simulink model "RL_TTS3_Controller_Blank_NLC_valve_E"  (R2019b)
settings: Solver=FixedStepAuto  StartTime=0.0  StopTime=600  FixedStep=0.01  RelTol=1e-3
PostLoadFcn:
  | if any(exist('dsrtsu_mdlpostloadfcn', 'file') ~= 0), dsrtsu_mdlpostloadfcn('Execute', bdroot); end
values from neighbouring files (symbols this model uses):
  Ts = 0.1    [RL_TTS3_Controller_Blank.mat]
libraries: simulink x2
settings Model: DSRTSU_INTERNAL_RTI_VER=550  DSRTSU_INTERNAL_RTI_TYPE=rti1104  RTICANMMDATA=struct('GeneralSetupData',struct('modelroot','E:\Will\RemoteLabs\TTS3\HostPC','generalsettings',struct('filesettings',struct('destfolder',struct('Name','RTICANMM_FILES','Check',1),'buildfolder',struct('Name','.','Check',1),'AbsDestfolder',struct('Name','E:\Will\RemoteLabs\TTS3\HostPC\RTICANMM_FILES'),'AbsBuildfolder',struct('Name','E:\Will\RemoteLabs\TTS3\HostPC'))),'options',struct('addpaths',1,'rmpaths',1,'addtrcexclusion',true,'cannavigator',struct('checkmonitoring',0),'show_usrtrc',0,'use_usrtrc',0),'advanced',struct('options',ones(1,100)),'MPSetup',{{}},'RTI',struct('Type','RTI1104','Ver','7.13','Date','02-Nov-2019'),'modelname','TTS3_Controller_Test_OL','block','TTS3_Controller_Test_OL'))  DSRTSU_INTERNAL_RTIFPGA=150  Creator=whendrix  LastModifiedBy=karan
settings OptimizationCC: BlockReduction=off  OptimizeBlockIOStorage=off  BufferReuse=off  GlobalBufferReuse=off  ExpressionFolding=off  LocalBlockOutputs=off  OptimizeDataStoreBuffers=off  BusAssignmentInplaceUpdate=off
settings DebuggingCC: BusObjectLabelMismatch=none
settings HardwareCC: ProdBitPerPointer=32  ProdBitPerSizeT=32  ProdBitPerPtrDiffT=32  ProdLargestAtomicInteger=Integer  ProdEndianess=BigEndian  ProdWordSize=32  ProdHWDeviceType=Custom Processor->Custom  TargetIntDivRoundTo=Zero  TargetEndianess=BigEndian  TargetHWDeviceType=Custom Processor->Custom
settings ModelReferenceCC: ModelReferenceNumInstancesAllowed=Single  ModelReferenceMinAlgLoopOccurrences=on
settings SFSimCC: MATLABDynamicMemAlloc=off  CustomCodeUndefinedFunction=UseInterfaceOnly
settings RTWCC: Description=dSPACE DS1104 Hardware Platform  SystemTargetFile=rti1104.tlc  MakeCommand=make_rti  TemplateMakefile=rti1104.tmf
settings CodeAppCC: MaxIdLength=63
settings STFCustomTargetCC: ParMdlRefBuildCompliant=on  SystemTargetFile=rti1104.tlc
settings GRTTargetCC: TargetLangStandard=C89/C90 (ANSI)  CompOptLevelCompliant=off  ConcurrentExecutionCompliant=off  CombineOutputUpdateFcns=off  MatFileLogging=off  CPPClassGenCompliant=off  UseToolchainInfoCompliant=off

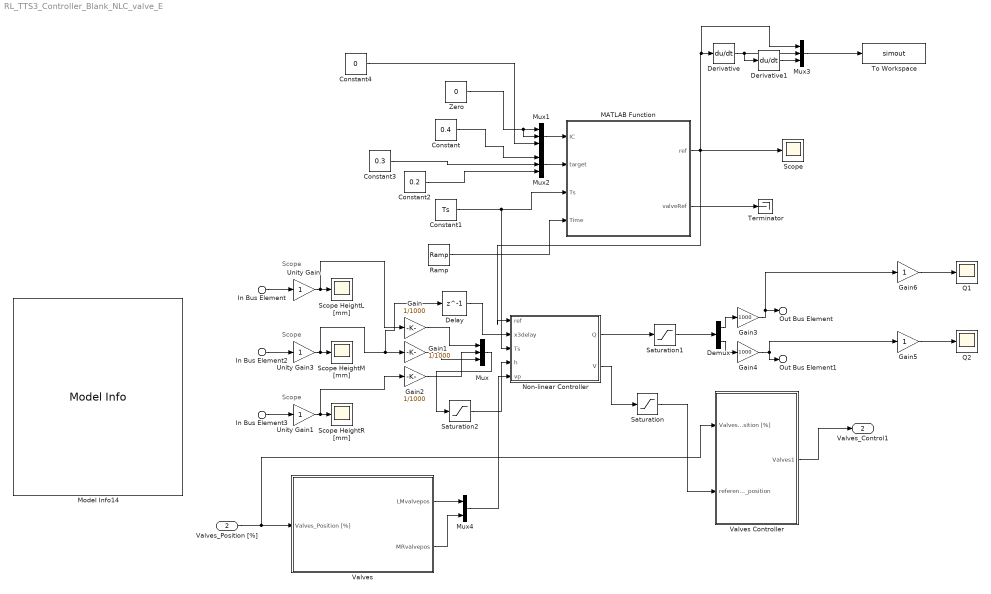
== system RL_TTS3_Controller_Blank_NLC_valve_E ==
  note: Scope
  note: Scope
  note: Scope
  In Bus Element : Inport  PortName=Heights [mm]  Element=Left
  In Bus Element2 : Inport  PortName=Heights [mm]  Element=Middle
  In Bus Element3 : Inport  PortName=Heights [mm]  Element=Right
  Valves_Position [%] : Inport  Port=2  OutDataTypeStr=Bus: ValvesSOCI
  Constant : Constant  Value=0.4
  Constant1 : Constant  Value=Ts
  Constant2 : Constant  Value=0.2
  Constant3 : Constant  Value=0.3
  Constant4 : Constant  Value=0
  Delay : Delay  DelayLength=1
  Demux : Demux  Outputs=2
  Derivative : Derivative
  Derivative1 : Derivative
  Gain : Gain  Gain=1/1000
  Gain1 : Gain  Gain=1/1000
  Gain2 : Gain  Gain=1/1000
  Gain3 : Gain  Gain=1000
  Gain4 : Gain  Gain=1000
  Gain5 : Gain
  Gain6 : Gain
  MATLAB Function : MATLAB Function  TreatAsAtomicUnit=on
  Model Info14 : simulink/Model-Wide Utilities/Model Info  Frame=on  DisplayStringWithTags=|  HorizontalTextAlignment=Left  LeftAlignmentValue=0.02
      | Start model for the "Three Tank"
      | experiment on the "Three Tank" setup.
      | Version: 1.0
      | 
      | 
      | INFORMATION
      | ----------------------
      | 
      | Unity Gain block before Scope is needed for
      | RemoteLabs compatebility. 
      | Do not modify or remove!
      | 
      | Pump range:
      | 0 to 0.102 [l/s]
      | 
      | The 5 Valves are labeled according 
      | to their position:
      | 
      |    LM  MR
      |      X     X
      |  X      X      X
      | LD    MD   RD
      | 
      | L = Left
      | M = Middle
      | R = Right
      | D = Down
  Mux{,1..3} (4 alike) : Mux  Inputs=3
  Mux4 : Mux  Inputs=2
  Non-linear Controller : MATLAB Function  TreatAsAtomicUnit=on
  Q1 : Scope
  Q2 : Scope
  Ramp : simulink/Sources/Ramp  slope=1  start=0  InitialOutput=0
  Saturation : Saturate  UpperLimit=100  LowerLimit=0
  Saturation1 : Saturate  UpperLimit=1.02e-4  LowerLimit=0
  Saturation2 : Saturate  UpperLimit=0.6  LowerLimit=0
  Scope : Scope
  Scope HeightL [mm] : Scope
  Scope HeightM [mm] : Scope
  Scope HeightR [mm] : Scope
  Terminator : Terminator
  To Workspace : ToWorkspace  VariableName=simout  SaveFormat=Timeseries  SampleTime=-1
  Unity Gain : Gain
  Unity Gain1 : Gain
  Unity Gain3 : Gain
  Valves : Subsystem  TreatAsAtomicUnit=on
  Valves Controller : Subsystem
  Zero : Constant  Value=0  OutDataTypeStr=Inherit: Inherit via back propagation
  Out Bus Element : Outport  VectorParamsAs1DForOutWhenUnconnected=off  PortName=Pumps [l/s]  Element=Left
  Out Bus Element1 : Outport  VectorParamsAs1DForOutWhenUnconnected=off  PortName=Pumps [l/s]  Element=Right
  Valves_Control1 : Outport  Port=2  OutDataTypeStr=Bus: ValvesSICO  VectorParamsAs1DForOutWhenUnconnected=off
  wires:
  Unity Gain/1 -> Gain/1, Scope HeightL [mm]/1
  Unity Gain3/1 -> Gain1/1, Delay/1, Scope HeightM [mm]/1
  Unity Gain1/1 -> Gain2/1, Scope HeightR [mm]/1
  In Bus Element/1 -> Unity Gain/1
  In Bus Element2/1 -> Unity Gain3/1
  In Bus Element3/1 -> Unity Gain1/1
  Mux/1 -> Saturation2/1
  Gain2/1 -> Mux/2
  Gain1/1 -> Mux/3
  Gain/1 -> Mux/1
  Saturation1/1 -> Demux/1
  Gain3/1 -> Gain6/1, Out Bus Element/1
  Demux/1 -> Gain3/1
  Demux/2 -> Gain4/1
  Gain4/1 -> Gain5/1, Out Bus Element1/1
  Valves Controller/1(Valves1) -> Valves_Control1/1
  Saturation/1 -> Valves Controller/2("reference_valve_position ")
  Mux1/1 -> MATLAB Function/1(IC)
  Mux3/1 -> To Workspace/1
  Constant/1 -> Mux2/1
  MATLAB Function/1(ref) -> Non-linear Controller/1(ref), Scope/1, Mux3/1, Derivative/1
  Constant4/1 -> Mux1/3
  MATLAB Function/2(valveRef) -> Terminator/1
  Constant3/1 -> Mux2/2
  Zero/1 -> Mux1/2, Mux1/1
  Derivative1/1 -> Mux3/3
  Constant1/1 -> Non-linear Controller/3(Ts), MATLAB Function/3(Ts)
  Constant2/1 -> Mux2/3
  Derivative/1 -> Derivative1/1, Mux3/2
  Mux2/1 -> MATLAB Function/2(target)
  Ramp/1 -> MATLAB Function/4(Time)
  Gain5/1 -> Q2/1
  Gain6/1 -> Q1/1
  Delay/1 -> Non-linear Controller/2(x3delay)
  Non-linear Controller/2(V) -> Saturation/1
  Valves_Position [%]/1 -> Valves Controller/1(Valves_Position [%]), Valves/1(Valves_Position [%])
  Valves/1(LMvalvepos) -> Mux4/1
  Valves/2("MRvalvepos ") -> Mux4/2
  Mux4/1 -> Non-linear Controller/5(vp)
  Non-linear Controller/1(Q) -> Saturation1/1
  Saturation2/1 -> Non-linear Controller/4(h)

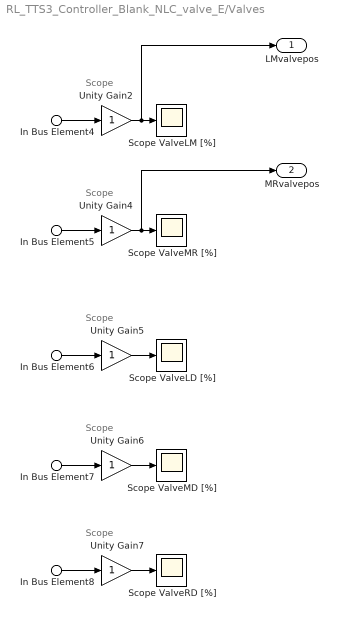
== system RL_TTS3_Controller_Blank_NLC_valve_E/Valves ==
  note: Scope
  note: Scope
  note: Scope
  note: Scope
  note: Scope
  In Bus Element4 : Inport  PortName=Valves_Position [%]  Element=LeftMiddle
  In Bus Element5 : Inport  PortName=Valves_Position [%]  Element=MiddleRight
  In Bus Element6 : Inport  PortName=Valves_Position [%]  Element=LeftDown
  In Bus Element7 : Inport  PortName=Valves_Position [%]  Element=MiddleDown
  In Bus Element8 : Inport  PortName=Valves_Position [%]  Element=RightDown
  Scope ValveLD [%] : Scope
  Scope ValveLM [%] : Scope
  Scope ValveMD [%] : Scope
  Scope ValveMR [%] : Scope
  Scope ValveRD [%] : Scope
  Unity Gain{2,4..7} (5 alike) : Gain
  LMvalvepos : Outport
  "MRvalvepos " : Outport  Port=2
  wires:
  In Bus Element5/1 -> Unity Gain4/1
  In Bus Element4/1 -> Unity Gain2/1
  In Bus Element7/1 -> Unity Gain6/1
  Unity Gain6/1 -> Scope ValveMD [%]/1
  In Bus Element6/1 -> Unity Gain5/1
  In Bus Element8/1 -> Unity Gain7/1
  Unity Gain7/1 -> Scope ValveRD [%]/1
  Unity Gain4/1 -> "MRvalvepos "/1, Scope ValveMR [%]/1
  Unity Gain5/1 -> Scope ValveLD [%]/1
  Unity Gain2/1 -> LMvalvepos/1, Scope ValveLM [%]/1

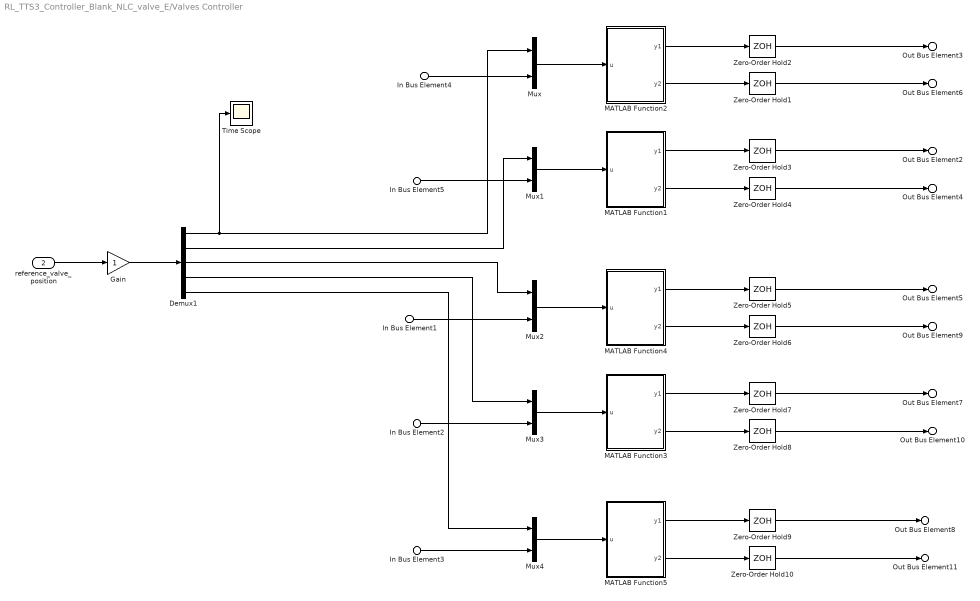
== system RL_TTS3_Controller_Blank_NLC_valve_E/Valves Controller ==
  In Bus Element4 : Inport  PortName=Valves_Position [%]  Element=LeftMiddle
  In Bus Element5 : Inport  PortName=Valves_Position [%]  Element=MiddleRight
  In Bus Element1 : Inport  PortName=Valves_Position [%]  Element=LeftDown
  In Bus Element2 : Inport  PortName=Valves_Position [%]  Element=MiddleDown
  In Bus Element3 : Inport  PortName=Valves_Position [%]  Element=RightDown
  "reference_valve_position " : Inport  Port=2
  Demux1 : Demux  Outputs=5
  Gain : Gain
  MATLAB Function1 : MATLAB Function  TreatAsAtomicUnit=on
  MATLAB Function2 : MATLAB Function  TreatAsAtomicUnit=on
  MATLAB Function3 : MATLAB Function  TreatAsAtomicUnit=on
  MATLAB Function4 : MATLAB Function  TreatAsAtomicUnit=on
  MATLAB Function5 : MATLAB Function  TreatAsAtomicUnit=on
  Mux{,1..4} (5 alike) : Mux  Inputs=2
  Time Scope : Scope
  Zero-Order Hold{1..10} (10 alike) : ZeroOrderHold  SampleTime=0.5
  Out Bus Element8 : Outport  VectorParamsAs1DForOutWhenUnconnected=off  PortName=Valves1  Element=RightDown.Open
  Out Bus Element11 : Outport  VectorParamsAs1DForOutWhenUnconnected=off  PortName=Valves1  Element=RightDown.Close
  Out Bus Element5 : Outport  VectorParamsAs1DForOutWhenUnconnected=off  PortName=Valves1  Element=LeftDown.Open
  Out Bus Element9 : Outport  VectorParamsAs1DForOutWhenUnconnected=off  PortName=Valves1  Element=LeftDown.Close
  Out Bus Element7 : Outport  VectorParamsAs1DForOutWhenUnconnected=off  PortName=Valves1  Element=MiddleDown.Open
  Out Bus Element10 : Outport  VectorParamsAs1DForOutWhenUnconnected=off  PortName=Valves1  Element=MiddleDown.Close
  Out Bus Element2 : Outport  VectorParamsAs1DForOutWhenUnconnected=off  PortName=Valves1  Element=MiddleRight.Open
  Out Bus Element4 : Outport  VectorParamsAs1DForOutWhenUnconnected=off  PortName=Valves1  Element=MiddleRight.Close
  Out Bus Element3 : Outport  VectorParamsAs1DForOutWhenUnconnected=off  PortName=Valves1  Element=LeftMiddle.Open
  Out Bus Element6 : Outport  VectorParamsAs1DForOutWhenUnconnected=off  PortName=Valves1  Element=LeftMiddle.Close
  wires:
  Zero-Order Hold5/1 -> Out Bus Element5/1
  Zero-Order Hold6/1 -> Out Bus Element9/1
  Zero-Order Hold9/1 -> Out Bus Element8/1
  Zero-Order Hold10/1 -> Out Bus Element11/1
  Zero-Order Hold8/1 -> Out Bus Element10/1
  Zero-Order Hold7/1 -> Out Bus Element7/1
  In Bus Element4/1 -> Mux/2
  Mux/1 -> MATLAB Function2/1(u)
  In Bus Element5/1 -> Mux1/2
  Demux1/2 -> Mux1/1
  Zero-Order Hold1/1 -> Out Bus Element6/1
  Zero-Order Hold2/1 -> Out Bus Element3/1
  Demux1/1 -> Time Scope/1, Mux/1
  Mux1/1 -> MATLAB Function1/1(u)
  Zero-Order Hold3/1 -> Out Bus Element2/1
  Zero-Order Hold4/1 -> Out Bus Element4/1
  Mux3/1 -> MATLAB Function3/1(u)
  Demux1/3 -> Mux2/1
  Demux1/4 -> Mux3/1
  In Bus Element2/1 -> Mux3/2
  Mux2/1 -> MATLAB Function4/1(u)
  In Bus Element1/1 -> Mux2/2
  In Bus Element3/1 -> Mux4/2
  Demux1/5 -> Mux4/1
  Mux4/1 -> MATLAB Function5/1(u)
  "reference_valve_position "/1 -> Gain/1
  Gain/1 -> Demux1/1
  MATLAB Function2/1(y1) -> Zero-Order Hold2/1
  MATLAB Function2/2(y2) -> Zero-Order Hold1/1
  MATLAB Function1/1(y1) -> Zero-Order Hold3/1
  MATLAB Function1/2(y2) -> Zero-Order Hold4/1
  MATLAB Function4/1(y1) -> Zero-Order Hold5/1
  MATLAB Function4/2(y2) -> Zero-Order Hold6/1
  MATLAB Function3/1(y1) -> Zero-Order Hold7/1
  MATLAB Function3/2(y2) -> Zero-Order Hold8/1
  MATLAB Function5/1(y1) -> Zero-Order Hold9/1
  MATLAB Function5/2(y2) -> Zero-Order Hold10/1

== matlab function RL_TTS3_Controller_Blank_NLC_valve_E/Valves Controller/MATLAB Function2 ==
  data: u input; y1 output; y2 output
function [y1,y2] = fcn(u)
    if u(2)>u(1)
        y1 = false;
        y2 = true;
    elseif u(1)>u(2)
        y1 = true;
        y2 = false;
    else
        y1 = false;
        y2 = false;
    end
end

== matlab function RL_TTS3_Controller_Blank_NLC_valve_E/Non-linear Controller ==
  data: ref input; x3delay input; Ts input; h input; Q output; V output; vp input
function [Q,V] = fcn(ref,x3delay,Ts,h,vp)

xr = [0.2 0.3 0.25];
x3dot = (h(3)-x3delay)/Ts;
% xr = [ref(1) ref(2) ref(3)];
A = 0.0154; S = 5e-5; g = 9.81;
x1 = h(1); x2 = h(2); x3 = h(3); x4 = vp(1); x5 = vp(2); g = 9.81; 
c1 = 16.1462; c2 = 15.5166; cc = 12/100; cd = 100/99;
x1r = xr(1); x2r = xr(2); x3r = xr(3);

Q = [0 0];
V = zeros(1,5);

u1 = A*(x1r - x1 + (2^(1/2)*S*c1*g^(1/2)*exp(cc*x4)*(x1 - x3))/(A*abs(x1 - x3)^(1/2)*(exp(cc*x4) + 1)));
u2 = A*(x2r - x2 + (2^(1/2)*S*c2*g^(1/2)*exp(cc*x5)*(x2 - x3))/(A*abs(x2 - x3)^(1/2)*(exp(cc*x5) + 1)));
u3 = (2^(1/2)*A*c1*sign(x1 - x3)^2*sign(x2 - x3)^2*exp(cc*x4)*sign(g)*(x1 - x3)*(exp(cc*x4) + 1)^2*(exp(cc*x5) + 1)^4*(x3r - 2*x3dot - x2 + (((2^(1/2)*S*c1*g^(1/2)*exp(cc*x4)*sign(g))/(2*abs(x1 - x3)^(1/2)*(exp(cc*x4) + 1)) + (2^(1/2)*S*c2*g^(1/2)*exp(cc*x5)*sign(g))/(2*abs(x2 - x3)^(1/2)*(exp(cc*x5) + 1)))*((2^(1/2)*S*c1*g^(1/2)*exp(cc*x4)*sign(g)*(x1 - x3))/(abs(x1 - x3)^(1/2)*(exp(cc*x4) + 1)) + (2^(1/2)*S*c2*g^(1/2)*exp(cc*x5)*sign(g)*(x2 - x3))/(abs(x2 - x3)^(1/2)*(exp(cc*x5) + 1))))/A^2 + (S^2*c1^2*g*sign(x1 - x3)*exp(2*cc*x4))/(A^2*(exp(cc*x4) + 1)^2) + (S^2*c2^2*g*sign(x2 - x3)*exp(2*cc*x5))/(A^2*(exp(cc*x5) + 1)^2) + (2^(1/2)*S*c1*cc*cd*g^(1/2)*x4*exp(cc*x4)*sign(g)*(x1 - x3))/(A^2*abs(x1 - x3)^(1/2)*(exp(cc*x4) + 1)^2) + (2^(1/2)*S*c2*cc*cd*g^(1/2)*x5*exp(cc*x5)*sign(g)*(x2 - x3))/(A^2*abs(x2 - x3)^(1/2)*(exp(cc*x5) + 1)^2)))/(2*S*cc*cd*g^(1/2)*abs(x1 - x3)^(1/2)*(6*c1^2*x1*sign(x1 - x3)*exp(2*cc*(x4 + x5)) - 6*c1^2*x3*sign(x1 - x3)*exp(2*cc*(x4 + x5)) + 6*c2^2*x2*sign(x2 - x3)*exp(2*cc*(x4 + x5)) - 6*c2^2*x3*sign(x2 - x3)*exp(2*cc*(x4 + x5)) + c1^2*x1*sign(x1 - x3)*exp(2*cc*x4) - c1^2*x3*sign(x1 - x3)*exp(2*cc*x4) + c2^2*x2*sign(x2 - x3)*exp(2*cc*x5) - c2^2*x3*sign(x2 - x3)*exp(2*cc*x5) + 4*c1^2*x1*sign(x1 - x3)*exp(cc*(2*x4 + x5)) + c1^2*x1*sign(x1 - x3)*exp(2*cc*(x4 + 2*x5)) - 4*c1^2*x3*sign(x1 - x3)*exp(cc*(2*x4 + x5)) + 4*c2^2*x2*sign(x2 - x3)*exp(cc*(x4 + 2*x5)) - c1^2*x3*sign(x1 - x3)*exp(2*cc*(x4 + 2*x5)) - 4*c2^2*x3*sign(x2 - x3)*exp(cc*(x4 + 2*x5)) + c2^2*x2*sign(x2 - x3)*exp(2*cc*(2*x4 + x5)) - c2^2*x3*sign(x2 - x3)*exp(2*cc*(2*x4 + x5)) + 4*c1^2*x1*sign(x1 - x3)*exp(cc*(2*x4 + 3*x5)) - 4*c1^2*x3*sign(x1 - x3)*exp(cc*(2*x4 + 3*x5)) + 4*c2^2*x2*sign(x2 - x3)*exp(cc*(3*x4 + 2*x5)) - 4*c2^2*x3*sign(x2 - x3)*exp(cc*(3*x4 + 2*x5)))) - (c1*c2*sign(x1 - x3)^2*sign(x2 - x3)^2*exp(cc*x4)*exp(cc*x5)*(x1 - x3)*(exp(cc*x4) + 1)^2*(exp(cc*x5) + 1)^3*(x2r - x2 + (2^(1/2)*S*c2*g^(1/2)*exp(cc*x5)*(x2 - x3))/(A*abs(x2 - x3)^(1/2)*(exp(cc*x5) + 1))))/(2*cc*cd*abs(x1 - x3)^(1/2)*abs(x2 - x3)^(1/2)*(6*c1^2*x1*sign(x1 - x3)*exp(2*cc*(x4 + x5)) - 6*c1^2*x3*sign(x1 - x3)*exp(2*cc*(x4 + x5)) + 6*c2^2*x2*sign(x2 - x3)*exp(2*cc*(x4 + x5)) - 6*c2^2*x3*sign(x2 - x3)*exp(2*cc*(x4 + x5)) + c1^2*x1*sign(x1 - x3)*exp(2*cc*x4) - c1^2*x3*sign(x1 - x3)*exp(2*cc*x4) + c2^2*x2*sign(x2 - x3)*exp(2*cc*x5) - c2^2*x3*sign(x2 - x3)*exp(2*cc*x5) + 4*c1^2*x1*sign(x1 - x3)*exp(cc*(2*x4 + x5)) + c1^2*x1*sign(x1 - x3)*exp(2*cc*(x4 + 2*x5)) - 4*c1^2*x3*sign(x1 - x3)*exp(cc*(2*x4 + x5)) + 4*c2^2*x2*sign(x2 - x3)*exp(cc*(x4 + 2*x5)) - c1^2*x3*sign(x1 - x3)*exp(2*cc*(x4 + 2*x5)) - 4*c2^2*x3*sign(x2 - x3)*exp(cc*(x4 + 2*x5)) + c2^2*x2*sign(x2 - x3)*exp(2*cc*(2*x4 + x5)) - c2^2*x3*sign(x2 - x3)*exp(2*cc*(2*x4 + x5)) + 4*c1^2*x1*sign(x1 - x3)*exp(cc*(2*x4 + 3*x5)) - 4*c1^2*x3*sign(x1 - x3)*exp(cc*(2*x4 + 3*x5)) + 4*c2^2*x2*sign(x2 - x3)*exp(cc*(3*x4 + 2*x5)) - 4*c2^2*x3*sign(x2 - x3)*exp(cc*(3*x4 + 2*x5)))) - (c1^2*sign(x1 - x3)^3*sign(x2 - x3)^2*exp(2*cc*x4)*(exp(cc*x4) + 1)*(exp(cc*x5) + 1)^4*(x1r - x1 + (2^(1/2)*S*c1*g^(1/2)*exp(cc*x4)*(x1 - x3))/(A*((x1 - x3)/sign(x1 - x3))^(1/2)*(exp(cc*x4) + 1))))/(2*cc*cd*(6*c1^2*x1*sign(x1 - x3)*exp(2*cc*(x4 + x5)) - 6*c1^2*x3*sign(x1 - x3)*exp(2*cc*(x4 + x5)) + 6*c2^2*x2*sign(x2 - x3)*exp(2*cc*(x4 + x5)) - 6*c2^2*x3*sign(x2 - x3)*exp(2*cc*(x4 + x5)) + c1^2*x1*sign(x1 - x3)*exp(2*cc*x4) - c1^2*x3*sign(x1 - x3)*exp(2*cc*x4) + c2^2*x2*sign(x2 - x3)*exp(2*cc*x5) - c2^2*x3*sign(x2 - x3)*exp(2*cc*x5) + 4*c1^2*x1*sign(x1 - x3)*exp(cc*(2*x4 + x5)) + c1^2*x1*sign(x1 - x3)*exp(2*cc*(x4 + 2*x5)) - 4*c1^2*x3*sign(x1 - x3)*exp(cc*(2*x4 + x5)) + 4*c2^2*x2*sign(x2 - x3)*exp(cc*(x4 + 2*x5)) - c1^2*x3*sign(x1 - x3)*exp(2*cc*(x4 + 2*x5)) - 4*c2^2*x3*sign(x2 - x3)*exp(cc*(x4 + 2*x5)) + c2^2*x2*sign(x2 - x3)*exp(2*cc*(2*x4 + x5)) - c2^2*x3*sign(x2 - x3)*exp(2*cc*(2*x4 + x5)) + 4*c1^2*x1*sign(x1 - x3)*exp(cc*(2*x4 + 3*x5)) - 4*c1^2*x3*sign(x1 - x3)*exp(cc*(2*x4 + 3*x5)) + 4*c2^2*x2*sign(x2 - x3)*exp(cc*(3*x4 + 2*x5)) - 4*c2^2*x3*sign(x2 - x3)*exp(cc*(3*x4 + 2*x5))));
u4 = (2^(1/2)*A*c2*sign(x1 - x3)^2*sign(x2 - x3)^2*exp(cc*x5)*sign(g)*(x2 - x3)*(exp(cc*x4) + 1)^4*(exp(cc*x5) + 1)^2*(x3r - 2*x3dot - x2 + (((2^(1/2)*S*c1*g^(1/2)*exp(cc*x4)*sign(g))/(2*abs(x1 - x3)^(1/2)*(exp(cc*x4) + 1)) + (2^(1/2)*S*c2*g^(1/2)*exp(cc*x5)*sign(g))/(2*abs(x2 - x3)^(1/2)*(exp(cc*x5) + 1)))*((2^(1/2)*S*c1*g^(1/2)*exp(cc*x4)*sign(g)*(x1 - x3))/(abs(x1 - x3)^(1/2)*(exp(cc*x4) + 1)) + (2^(1/2)*S*c2*g^(1/2)*exp(cc*x5)*sign(g)*(x2 - x3))/(abs(x2 - x3)^(1/2)*(exp(cc*x5) + 1))))/A^2 + (S^2*c1^2*g*sign(x1 - x3)*exp(2*cc*x4))/(A^2*(exp(cc*x4) + 1)^2) + (S^2*c2^2*g*sign(x2 - x3)*exp(2*cc*x5))/(A^2*(exp(cc*x5) + 1)^2) + (2^(1/2)*S*c1*cc*cd*g^(1/2)*x4*exp(cc*x4)*sign(g)*(x1 - x3))/(A^2*abs(x1 - x3)^(1/2)*(exp(cc*x4) + 1)^2) + (2^(1/2)*S*c2*cc*cd*g^(1/2)*x5*exp(cc*x5)*sign(g)*(x2 - x3))/(A^2*abs(x2 - x3)^(1/2)*(exp(cc*x5) + 1)^2)))/(2*S*cc*cd*g^(1/2)*abs(x2 - x3)^(1/2)*(6*c1^2*x1*sign(x1 - x3)*exp(2*cc*(x4 + x5)) - 6*c1^2*x3*sign(x1 - x3)*exp(2*cc*(x4 + x5)) + 6*c2^2*x2*sign(x2 - x3)*exp(2*cc*(x4 + x5)) - 6*c2^2*x3*sign(x2 - x3)*exp(2*cc*(x4 + x5)) + c1^2*x1*sign(x1 - x3)*exp(2*cc*x4) - c1^2*x3*sign(x1 - x3)*exp(2*cc*x4) + c2^2*x2*sign(x2 - x3)*exp(2*cc*x5) - c2^2*x3*sign(x2 - x3)*exp(2*cc*x5) + 4*c1^2*x1*sign(x1 - x3)*exp(cc*(2*x4 + x5)) + c1^2*x1*sign(x1 - x3)*exp(2*cc*(x4 + 2*x5)) - 4*c1^2*x3*sign(x1 - x3)*exp(cc*(2*x4 + x5)) + 4*c2^2*x2*sign(x2 - x3)*exp(cc*(x4 + 2*x5)) - c1^2*x3*sign(x1 - x3)*exp(2*cc*(x4 + 2*x5)) - 4*c2^2*x3*sign(x2 - x3)*exp(cc*(x4 + 2*x5)) + c2^2*x2*sign(x2 - x3)*exp(2*cc*(2*x4 + x5)) - c2^2*x3*sign(x2 - x3)*exp(2*cc*(2*x4 + x5)) + 4*c1^2*x1*sign(x1 - x3)*exp(cc*(2*x4 + 3*x5)) - 4*c1^2*x3*sign(x1 - x3)*exp(cc*(2*x4 + 3*x5)) + 4*c2^2*x2*sign(x2 - x3)*exp(cc*(3*x4 + 2*x5)) - 4*c2^2*x3*sign(x2 - x3)*exp(cc*(3*x4 + 2*x5)))) - (c1*c2*sign(x1 - x3)^2*sign(x2 - x3)^2*exp(cc*x4)*exp(cc*x5)*(x2 - x3)*(exp(cc*x4) + 1)^3*(exp(cc*x5) + 1)^2*(x1r - x1 + (2^(1/2)*S*c1*g^(1/2)*exp(cc*x4)*(x1 - x3))/(A*abs(x1 - x3)^(1/2)*(exp(cc*x4) + 1))))/(2*cc*cd*abs(x1 - x3)^(1/2)*abs(x2 - x3)^(1/2)*(6*c1^2*x1*sign(x1 - x3)*exp(2*cc*(x4 + x5)) - 6*c1^2*x3*sign(x1 - x3)*exp(2*cc*(x4 + x5)) + 6*c2^2*x2*sign(x2 - x3)*exp(2*cc*(x4 + x5)) - 6*c2^2*x3*sign(x2 - x3)*exp(2*cc*(x4 + x5)) + c1^2*x1*sign(x1 - x3)*exp(2*cc*x4) - c1^2*x3*sign(x1 - x3)*exp(2*cc*x4) + c2^2*x2*sign(x2 - x3)*exp(2*cc*x5) - c2^2*x3*sign(x2 - x3)*exp(2*cc*x5) + 4*c1^2*x1*sign(x1 - x3)*exp(cc*(2*x4 + x5)) + c1^2*x1*sign(x1 - x3)*exp(2*cc*(x4 + 2*x5)) - 4*c1^2*x3*sign(x1 - x3)*exp(cc*(2*x4 + x5)) + 4*c2^2*x2*sign(x2 - x3)*exp(cc*(x4 + 2*x5)) - c1^2*x3*sign(x1 - x3)*exp(2*cc*(x4 + 2*x5)) - 4*c2^2*x3*sign(x2 - x3)*exp(cc*(x4 + 2*x5)) + c2^2*x2*sign(x2 - x3)*exp(2*cc*(2*x4 + x5)) - c2^2*x3*sign(x2 - x3)*exp(2*cc*(2*x4 + x5)) + 4*c1^2*x1*sign(x1 - x3)*exp(cc*(2*x4 + 3*x5)) - 4*c1^2*x3*sign(x1 - x3)*exp(cc*(2*x4 + 3*x5)) + 4*c2^2*x2*sign(x2 - x3)*exp(cc*(3*x4 + 2*x5)) - 4*c2^2*x3*sign(x2 - x3)*exp(cc*(3*x4 + 2*x5)))) - (c2^2*sign(x1 - x3)^2*sign(x2 - x3)^3*exp(2*cc*x5)*(exp(cc*x4) + 1)^4*(exp(cc*x5) + 1)*(x2r - x2 + (2^(1/2)*S*c2*g^(1/2)*exp(cc*x5)*(x2 - x3))/(A*((x2 - x3)/sign(x2 - x3))^(1/2)*(exp(cc*x5) + 1))))/(2*cc*cd*(6*c1^2*x1*sign(x1 - x3)*exp(2*cc*(x4 + x5)) - 6*c1^2*x3*sign(x1 - x3)*exp(2*cc*(x4 + x5)) + 6*c2^2*x2*sign(x2 - x3)*exp(2*cc*(x4 + x5)) - 6*c2^2*x3*sign(x2 - x3)*exp(2*cc*(x4 + x5)) + c1^2*x1*sign(x1 - x3)*exp(2*cc*x4) - c1^2*x3*sign(x1 - x3)*exp(2*cc*x4) + c2^2*x2*sign(x2 - x3)*exp(2*cc*x5) - c2^2*x3*sign(x2 - x3)*exp(2*cc*x5) + 4*c1^2*x1*sign(x1 - x3)*exp(cc*(2*x4 + x5)) + c1^2*x1*sign(x1 - x3)*exp(2*cc*(x4 + 2*x5)) - 4*c1^2*x3*sign(x1 - x3)*exp(cc*(2*x4 + x5)) + 4*c2^2*x2*sign(x2 - x3)*exp(cc*(x4 + 2*x5)) - c1^2*x3*sign(x1 - x3)*exp(2*cc*(x4 + 2*x5)) - 4*c2^2*x3*sign(x2 - x3)*exp(cc*(x4 + 2*x5)) + c2^2*x2*sign(x2 - x3)*exp(2*cc*(2*x4 + x5)) - c2^2*x3*sign(x2 - x3)*exp(2*cc*(2*x4 + x5)) + 4*c1^2*x1*sign(x1 - x3)*exp(cc*(2*x4 + 3*x5)) - 4*c1^2*x3*sign(x1 - x3)*exp(cc*(2*x4 + 3*x5)) + 4*c2^2*x2*sign(x2 - x3)*exp(cc*(3*x4 + 2*x5)) - 4*c2^2*x3*sign(x2 - x3)*exp(cc*(3*x4 + 2*x5))));

% u1 = A*(x1r - x1 + (2^(1/2)*S*g^(1/2)*x4*(x1 - x3))/(A*abs(x1 - x3)^(1/2)));
% u2 = A*(x2r - x2 + (2^(1/2)*S*g^(1/2)*x5*(x2 - x3))/(A*abs(x2 - x3)^(1/2)));
% u3 = (9*2^(1/2)*A*abs(x1 - x3)^(1/2)*sign(x1 - x3)*sign(x2 - x3)^2*sign(g)*(x3r - 2*x3dot - x2 + (S^2*g*x4^2*sign(x1 - x3))/A^2 + (S^2*g*x5^2*sign(x2 - x3))/A^2 + (2^(1/2)*S*g^(1/2)*sign(g)*(x4*abs(x2 - x3)^(1/2) + x5*abs(x1 - x3)^(1/2))*((2^(1/2)*S*g^(1/2)*x4*sign(g)*(x1 - x3))/abs(x1 - x3)^(1/2) + (2^(1/2)*S*g^(1/2)*x5*sign(g)*(x2 - x3))/abs(x2 - x3)^(1/2)))/(2*A^2*abs(x1 - x3)^(1/2)*abs(x2 - x3)^(1/2)) + (2^(1/2)*S*cd*g^(1/2)*x4*sign(g)*(x1 - x3))/(A^2*abs(x1 - x3)^(1/2)) + (2^(1/2)*S*cd*g^(1/2)*x5*sign(g)*(x2 - x3))/(A^2*abs(x2 - x3)^(1/2))))/(200*S*g^(1/2)*(x1*sign(x1 - x3) + x2*sign(x2 - x3) - x3*sign(x1 - x3) - x3*sign(x2 - x3))) - (9*x5*abs(x1 - x3)^(1/2)*sign(x1 - x3)*sign(x2 - x3)^2*(x2r - x2 + (2^(1/2)*S*g^(1/2)*x5*(x2 - x3))/(A*abs(x2 - x3)^(1/2))))/(200*abs(x2 - x3)^(1/2)*(x1*sign(x1 - x3) + x2*sign(x2 - x3) - x3*sign(x1 - x3) - x3*sign(x2 - x3))) - (9*x4*sign(x1 - x3)^3*sign(x2 - x3)^2*(x1r - x1 + (2^(1/2)*S*g^(1/2)*x4*(x1 - x3))/(A*abs(x1 - x3)^(1/2))))/(200*(x1*sign(x1 - x3) + x2*sign(x2 - x3) - x3*sign(x1 - x3) - x3*sign(x2 - x3)));
% u4 = (9*2^(1/2)*A*abs(x2 - x3)^(1/2)*sign(x1 - x3)^2*sign(x2 - x3)*sign(g)*(x3r - 2*x3dot - x2 + (S^2*g*x4^2*sign(x1 - x3))/A^2 + (S^2*g*x5^2*sign(x2 - x3))/A^2 + (2^(1/2)*S*g^(1/2)*sign(g)*(x4*abs(x2 - x3)^(1/2) + x5*abs(x1 - x3)^(1/2))*((2^(1/2)*S*g^(1/2)*x4*sign(g)*(x1 - x3))/abs(x1 - x3)^(1/2) + (2^(1/2)*S*g^(1/2)*x5*sign(g)*(x2 - x3))/abs(x2 - x3)^(1/2)))/(2*A^2*abs(x1 - x3)^(1/2)*abs(x2 - x3)^(1/2)) + (2^(1/2)*S*cd*g^(1/2)*x4*sign(g)*(x1 - x3))/(A^2*abs(x1 - x3)^(1/2)) + (2^(1/2)*S*cd*g^(1/2)*x5*sign(g)*(x2 - x3))/(A^2*abs(x2 - x3)^(1/2))))/(200*S*g^(1/2)*(x1*sign(x1 - x3) + x2*sign(x2 - x3) - x3*sign(x1 - x3) - x3*sign(x2 - x3))) - (9*x4*abs(x2 - x3)^(1/2)*sign(x1 - x3)^2*sign(x2 - x3)*(x1r - x1 + (2^(1/2)*S*g^(1/2)*x4*(x1 - x3))/(A*abs(x1 - x3)^(1/2))))/(200*abs(x1 - x3)^(1/2)*(x1*sign(x1 - x3) + x2*sign(x2 - x3) - x3*sign(x1 - x3) - x3*sign(x2 - x3))) - (9*x5*sign(x1 - x3)^2*sign(x2 - x3)^3*(x2r - x2 + (2^(1/2)*S*g^(1/2)*x5*(x2 - x3))/(A*abs(x2 - x3)^(1/2))))/(200*(x1*sign(x1 - x3) + x2*sign(x2 - x3) - x3*sign(x1 - x3) - x3*sign(x2 - x3)));
if u1<0
    u1 = 0;
end
if u2<0
    u2 = 0;
end

Q(1) = u1;
Q(2) = u2;
V = [u3 u4 0 0 0];
end

== matlab function RL_TTS3_Controller_Blank_NLC_valve_E/Valves Controller/MATLAB Function1 ==
  data: u input; y1 output; y2 output
function [y1,y2] = fcn(u)
    if u(2)>u(1)
        y1 = false;
        y2 = true;
    elseif u(1)>u(2)
        y1 = true;
        y2 = false;
    else
        y1 = false;
        y2 = false;
    end
end

== matlab function RL_TTS3_Controller_Blank_NLC_valve_E/Valves Controller/MATLAB Function3 ==
  data: u input; y1 output; y2 output
function [y1,y2] = fcn(u)
    if u(2)>u(1)
        y1 = false;
        y2 = true;
    elseif u(1)>u(2)
        y1 = true;
        y2 = false;
    else
        y1 = false;
        y2 = false;
    end
end

== matlab function RL_TTS3_Controller_Blank_NLC_valve_E/Valves Controller/MATLAB Function4 ==
  data: u input; y1 output; y2 output
function [y1,y2] = fcn(u)
    if u(2)>u(1)
        y1 = false;
        y2 = true;
    elseif u(1)>u(2)
        y1 = true;
        y2 = false;
    else
        y1 = false;
        y2 = false;
    end
end

== matlab function RL_TTS3_Controller_Blank_NLC_valve_E/Valves Controller/MATLAB Function5 ==
  data: u input; y1 output; y2 output
function [y1,y2] = fcn(u)
    if u(2)>u(1)
        y1 = false;
        y2 = true;
    elseif u(1)>u(2)
        y1 = true;
        y2 = false;
    else
        y1 = false;
        y2 = false;
    end
end

== matlab function RL_TTS3_Controller_Blank_NLC_valve_E/MATLAB Function ==
  data: IC input; ref output; target input; valveRef output; Ts input; Time input
function [ref, valveRef] = fcn(IC, target,Ts,Time)
% input: IC, 3D vector of initial conditions of system
% input: target, 3D vector of target reference for fluid  heights
% input: Sampling time Ts

% output: ref, 3*1 vector containing fluid height references 
% output: valveRef, 2*1 vector containg valve references. Needed for MPC,
% can be ignored (use terminator block in simulink)

%% constants
Atank = 0.0154;
uMaxL = 0.1;        % from Bart's work
uMaxR =  0.09;      % from Bart's work
%% reshaping (check gode generation?)
IC = reshape(IC, [],1);             %  force IC to be a vector
target = reshape(target, [],1);     %  idem
%% calculations
tf = 1.1*sum(target)*Atank/(uMaxL+uMaxR-3*0.01)*1000;  % give a 10% margin for pump dynamics etc, choose 50% of maximum disturbance allowed as 'constant disturbance'
ref = zeros(3,1);
valveRef = zeros(2,1);
matr = [1 zeros(1,3);
        0 1  0    0;
        1 tf tf^2 tf^3;
        0 1 2*tf 3*tf^2];
invmatr = inv(matr);
if  Time < tf
    for i =1:3
        vec = [IC(i);0;target(i);0];
        polyCoeff = invmatr*vec;
        ref(i,1) = polyCoeff(1)+polyCoeff(2)*Time+polyCoeff(3)*Time.^2+polyCoeff(4)*Time.^3;
    end
else
    ref = target;
end
